simulink model "StandaloneDAQv07_R2014a"  (R2014a)
settings: Solver=FixedStepDiscrete  SolverMode=MultiTasking  StartTime=0.0  StopTime=inf  FixedStep=0.0005  RelTol=1e-3
values from neighbouring files (symbols this model uses):
  ANOMALY_INIT = 10    [DAQParams3_1ms_DDA.m]
  Calibration = getCalibrationParams_ATRIAS()    [DAQParams3_1ms_DDA.m]
  EnableFT = 0    [DAQParams3_1ms_DDA.m]
  EncoderAngleLimits = [60 240; 120 300; 60 240; 120 300; 60 240; 120 300; 60 240; 120 300; -30 30; -30 30; -inf inf; -inf inf; -inf inf; -inf inf; -30 30; -30 30; -inf inf; -90 90; -90 90]*pi/180    [DAQParams3_1ms_DDA.m]
  EncoderFiltSys = getDerivFilter(2, 5, 5, Ts)    [DAQParams3_1ms_DDA.m]
  EncoderThreshold = [5; 5; 5; 5; 5; 5; 5; 5; 5; 5; 250; 250; 250; 250; 5; 5; 5; 5; 5]*pi/180    [DAQParams3_1ms_DDA.m]
  IMUAngleLimits = [-180 180; -90 90; -90 90]*pi/180    [DAQParams3_1ms_DDA.m]
  IMUCommand = 70    [DAQParams3_1ms_DDA.m]
  IMUThreshold = 5*pi/180    (= 0.0872664625997)    [DAQParams3_1ms_DDA.m]
  MAX_ANOMALY = 30    [DAQParams3_1ms_DDA.m]
  MedullaCommand = 0    [DAQParams3_1ms_DDA.m]
  MicrostrainFiltSys = getDerivFilter(2, 5, 5, TsMicrostrain)    [DAQParams3_1ms_DDA.m]
  MODBUS_TIMEOUT = 0.02    [DAQParams3_1ms_DDA.m]
  ResetDAQ = 0    [DAQParams3_1ms_DDA.m]
  ResetYaw = 0    [DAQParams3_1ms_DDA.m]
  STREAMING_TIMEOUT = 0.1    [DAQParams3_1ms_DDA.m]
  TareFT = 0    [DAQParams3_1ms_DDA.m]
  Ts = 0.001    [DAQParams3_1ms_DDA.m]
  UseMicrostrainRate = 0    [DAQParams3_1ms_DDA.m]
undefined symbols (not defined in the file or in its folder): FTCalibration, GearOffset, IMUTorsoOffset, m_XR17D15x, standard
libraries: xpcethercatlib x167, speedgoatlib x13, dspswit3 x2, simulink x2, xpcseriallib x1, SpeedgoatModified x1
(part 2 of 4)

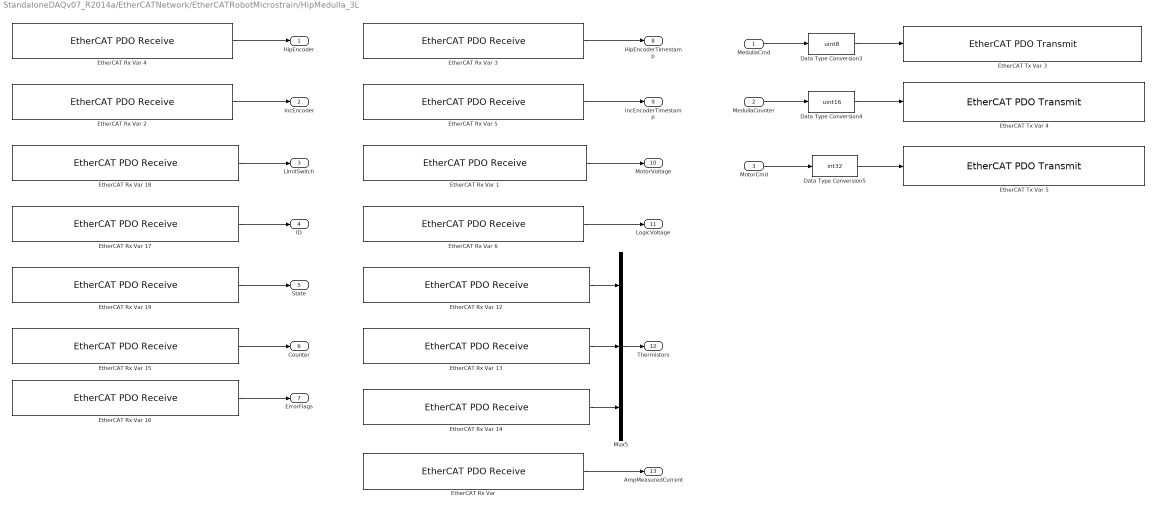
== system StandaloneDAQv07_R2014a/EtherCATNetwork/EtherCATRobotMicrostrain/HipMedulla_3L ==
  MedullaCmd : Inport
  MedullaCounter : Inport  Port=2
  MotorCmd : Inport  Port=3
  Data Type Conversion3 : DataTypeConversion  OutDataTypeStr=uint8  RndMeth=Simplest
  Data Type Conversion4 : DataTypeConversion  OutDataTypeStr=uint16  RndMeth=Simplest
  Data Type Conversion5 : DataTypeConversion  OutDataTypeStr=int32  RndMeth=Simplest
  "EtherCAT Rx Var " : xpcethercatlib/EtherCAT PDO Receive  Priority=2  sig_name=Box 6 (ATRIAS 2.1 Hip (Medulla 1.5)).Measured Current.Amp Measured Current  sig_offset=2480  sig_type=int16  type_size=16  sig_dim=1  device_id=0  sample_time=0.000500
  EtherCAT Rx Var 1 : xpcethercatlib/EtherCAT PDO Receive  Priority=2  sig_name=Box 6 (ATRIAS 2.1 Hip (Medulla 1.5)).Power.Motor Voltage  sig_offset=2400  sig_type=uint16  type_size=16  sig_dim=1  device_id=0  sample_time=0.000500
  EtherCAT Rx Var 12 : xpcethercatlib/EtherCAT PDO Receive  Priority=2  sig_name=Box 6 (ATRIAS 2.1 Hip (Medulla 1.5)).Thermistors.Thermistor 0  sig_offset=2432  sig_type=uint16  type_size=16  sig_dim=1  device_id=0  sample_time=0.000500
  EtherCAT Rx Var 13 : xpcethercatlib/EtherCAT PDO Receive  Priority=2  sig_name=Box 6 (ATRIAS 2.1 Hip (Medulla 1.5)).Thermistors.Thermistor 1  sig_offset=2448  sig_type=uint16  type_size=16  sig_dim=1  device_id=0  sample_time=0.000500
  EtherCAT Rx Var 14 : xpcethercatlib/EtherCAT PDO Receive  Priority=2  sig_name=Box 6 (ATRIAS 2.1 Hip (Medulla 1.5)).Thermistors.Thermistor 2  sig_offset=2464  sig_type=uint16  type_size=16  sig_dim=1  device_id=0  sample_time=0.000500
  EtherCAT Rx Var 15 : xpcethercatlib/EtherCAT PDO Receive  Priority=2  sig_name=Box 6 (ATRIAS 2.1 Hip (Medulla 1.5)).uController Status.Counter  sig_offset=2328  sig_type=uint8  type_size=8  sig_dim=1  device_id=0  sample_time=0.000500
  EtherCAT Rx Var 16 : xpcethercatlib/EtherCAT PDO Receive  Priority=2  sig_name=Box 6 (ATRIAS 2.1 Hip (Medulla 1.5)).uController Status.Error Flags  sig_offset=2336  sig_type=uint8  type_size=8  sig_dim=1  device_id=0  sample_time=0.000500
  EtherCAT Rx Var 17 : xpcethercatlib/EtherCAT PDO Receive  Priority=2  sig_name=Box 6 (ATRIAS 2.1 Hip (Medulla 1.5)).uController Status.ID  sig_offset=2312  sig_type=uint8  type_size=8  sig_dim=1  device_id=0  sample_time=0.000500
  EtherCAT Rx Var 18 : xpcethercatlib/EtherCAT PDO Receive  Priority=2  sig_name=Box 6 (ATRIAS 2.1 Hip (Medulla 1.5)).uController Status.Limit Switch  sig_offset=2344  sig_type=uint8  type_size=8  sig_dim=1  device_id=0  sample_time=0.000500
  EtherCAT Rx Var 19 : xpcethercatlib/EtherCAT PDO Receive  Priority=2  sig_name=Box 6 (ATRIAS 2.1 Hip (Medulla 1.5)).uController Status.State  sig_offset=2320  sig_type=uint8  type_size=8  sig_dim=1  device_id=0  sample_time=0.000500
  EtherCAT Rx Var 2 : xpcethercatlib/EtherCAT PDO Receive  Priority=2  sig_name=Box 6 (ATRIAS 2.1 Hip (Medulla 1.5)).Incremental Encoder.Incremental Encoder  sig_offset=2496  sig_type=uint16  type_size=16  sig_dim=1  device_id=0  sample_time=0.000500
  EtherCAT Rx Var 3 : xpcethercatlib/EtherCAT PDO Receive  Priority=2  sig_name=Box 6 (ATRIAS 2.1 Hip (Medulla 1.5)).Hip Encoder.Timestamp  sig_offset=2384  sig_type=uint16  type_size=16  sig_dim=1  device_id=0  sample_time=0.000500
  EtherCAT Rx Var 4 : xpcethercatlib/EtherCAT PDO Receive  Priority=2  sig_name=Box 6 (ATRIAS 2.1 Hip (Medulla 1.5)).Hip Encoder.Encoder  sig_offset=2352  sig_type=uint32  type_size=32  sig_dim=1  device_id=0  sample_time=0.000500
  EtherCAT Rx Var 5 : xpcethercatlib/EtherCAT PDO Receive  Priority=2  sig_name=Box 6 (ATRIAS 2.1 Hip (Medulla 1.5)).Incremental Encoder.Incremental Encoder Timestamp  sig_offset=2512  sig_type=uint16  type_size=16  sig_dim=1  device_id=0  sample_time=0.000500
  EtherCAT Rx Var 6 : xpcethercatlib/EtherCAT PDO Receive  Priority=2  sig_name=Box 6 (ATRIAS 2.1 Hip (Medulla 1.5)).Power.Logic Voltage  sig_offset=2416  sig_type=uint16  type_size=16  sig_dim=1  device_id=0  sample_time=0.000500
  EtherCAT Tx Var 3 : xpcethercatlib/EtherCAT PDO Transmit   Priority=3  sig_name=Box 6 (ATRIAS 2.1 Hip (Medulla 1.5)).uControllerInput.Command  sig_offset=2312  sig_type=uint8  type_size=8  sig_dim=1  device_id=0  sample_time=0.000500
  EtherCAT Tx Var 4 : xpcethercatlib/EtherCAT PDO Transmit   Priority=3  sig_name=Box 6 (ATRIAS 2.1 Hip (Medulla 1.5)).uControllerInput.Counter  sig_offset=2320  sig_type=uint16  type_size=16  sig_dim=1  device_id=0  sample_time=0.000500
  EtherCAT Tx Var 5 : xpcethercatlib/EtherCAT PDO Transmit   Priority=3  sig_name=Box 6 (ATRIAS 2.1 Hip (Medulla 1.5)).uControllerInput.Motor Current  sig_offset=2336  sig_type=int32  type_size=32  sig_dim=1  device_id=0  sample_time=0.000500
  Mux5 : Mux  Inputs=3
  HipEncoder : Outport
  IncEncoder : Outport  Port=2
  LimitSwitch : Outport  Port=3
  ID : Outport  Port=4
  State : Outport  Port=5
  Counter : Outport  Port=6
  ErrorFlags : Outport  Port=7
  HipEncoderTimestamp : Outport  Port=8
  IncEncoderTimestamp : Outport  Port=9
  MotorVoltage : Outport  Port=10
  LogicVoltage : Outport  Port=11
  Thermistors : Outport  Port=12
  AmpMeasuredCurrent : Outport  Port=13
  wires:
  Data Type Conversion3/1 -> EtherCAT Tx Var 3/1
  Data Type Conversion4/1 -> EtherCAT Tx Var 4/1
  Data Type Conversion5/1 -> EtherCAT Tx Var 5/1
  MedullaCmd/1 -> Data Type Conversion3/1
  MedullaCounter/1 -> Data Type Conversion4/1
  MotorCmd/1 -> Data Type Conversion5/1
  EtherCAT Rx Var 5/1 -> IncEncoderTimestamp/1
  EtherCAT Rx Var 4/1 -> HipEncoder/1
  EtherCAT Rx Var 3/1 -> HipEncoderTimestamp/1
  EtherCAT Rx Var 2/1 -> IncEncoder/1
  EtherCAT Rx Var 15/1 -> Counter/1
  EtherCAT Rx Var 17/1 -> ID/1
  EtherCAT Rx Var 18/1 -> LimitSwitch/1
  EtherCAT Rx Var 19/1 -> State/1
  EtherCAT Rx Var 16/1 -> ErrorFlags/1
  EtherCAT Rx Var 6/1 -> LogicVoltage/1
  EtherCAT Rx Var 1/1 -> MotorVoltage/1
  EtherCAT Rx Var 12/1 -> Mux5/1
  EtherCAT Rx Var 13/1 -> Mux5/2
  EtherCAT Rx Var 14/1 -> Mux5/3
  "EtherCAT Rx Var "/1 -> AmpMeasuredCurrent/1
  Mux5/1 -> Thermistors/1

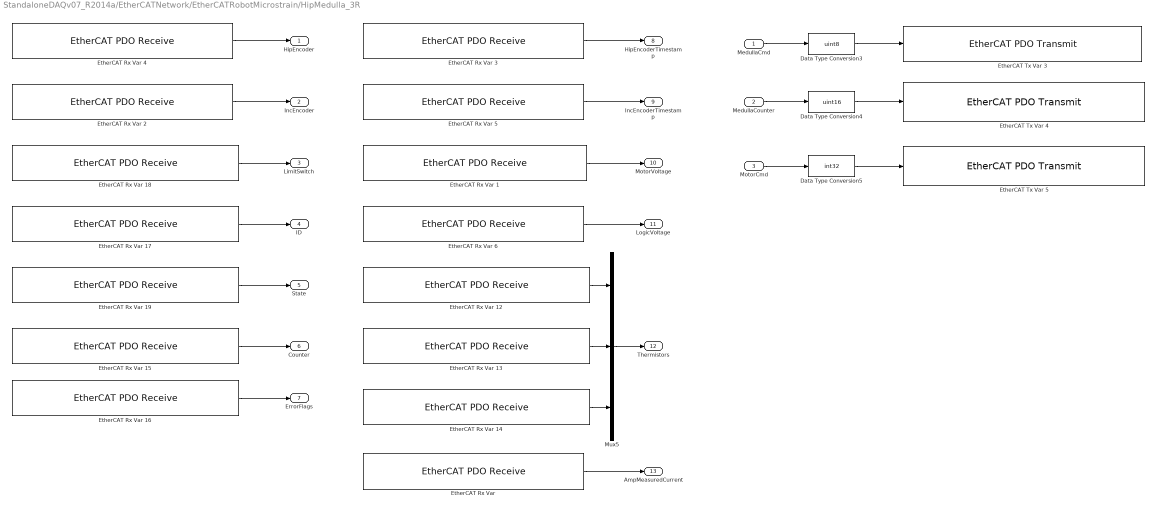
== system StandaloneDAQv07_R2014a/EtherCATNetwork/EtherCATRobotMicrostrain/HipMedulla_3R ==
  MedullaCmd : Inport
  MedullaCounter : Inport  Port=2
  MotorCmd : Inport  Port=3
  Data Type Conversion3 : DataTypeConversion  OutDataTypeStr=uint8  RndMeth=Simplest
  Data Type Conversion4 : DataTypeConversion  OutDataTypeStr=uint16  RndMeth=Simplest
  Data Type Conversion5 : DataTypeConversion  OutDataTypeStr=int32  RndMeth=Simplest
  "EtherCAT Rx Var " : xpcethercatlib/EtherCAT PDO Receive  Priority=2  sig_name=Box 5 (ATRIAS 2.1 Hip (Medulla 1.5)).Measured Current.Amp Measured Current  sig_offset=2264  sig_type=int16  type_size=16  sig_dim=1  device_id=0  sample_time=0.000500
  EtherCAT Rx Var 1 : xpcethercatlib/EtherCAT PDO Receive  Priority=2  sig_name=Box 5 (ATRIAS 2.1 Hip (Medulla 1.5)).Power.Motor Voltage  sig_offset=2184  sig_type=uint16  type_size=16  sig_dim=1  device_id=0  sample_time=0.000500
  EtherCAT Rx Var 12 : xpcethercatlib/EtherCAT PDO Receive  Priority=2  sig_name=Box 5 (ATRIAS 2.1 Hip (Medulla 1.5)).Thermistors.Thermistor 0  sig_offset=2216  sig_type=uint16  type_size=16  sig_dim=1  device_id=0  sample_time=0.000500
  EtherCAT Rx Var 13 : xpcethercatlib/EtherCAT PDO Receive  Priority=2  sig_name=Box 5 (ATRIAS 2.1 Hip (Medulla 1.5)).Thermistors.Thermistor 1  sig_offset=2232  sig_type=uint16  type_size=16  sig_dim=1  device_id=0  sample_time=0.000500
  EtherCAT Rx Var 14 : xpcethercatlib/EtherCAT PDO Receive  Priority=2  sig_name=Box 5 (ATRIAS 2.1 Hip (Medulla 1.5)).Thermistors.Thermistor 2  sig_offset=2248  sig_type=uint16  type_size=16  sig_dim=1  device_id=0  sample_time=0.000500
  EtherCAT Rx Var 15 : xpcethercatlib/EtherCAT PDO Receive  Priority=2  sig_name=Box 5 (ATRIAS 2.1 Hip (Medulla 1.5)).uController Status.Counter  sig_offset=2112  sig_type=uint8  type_size=8  sig_dim=1  device_id=0  sample_time=0.000500
  EtherCAT Rx Var 16 : xpcethercatlib/EtherCAT PDO Receive  Priority=2  sig_name=Box 5 (ATRIAS 2.1 Hip (Medulla 1.5)).uController Status.Error Flags  sig_offset=2120  sig_type=uint8  type_size=8  sig_dim=1  device_id=0  sample_time=0.000500
  EtherCAT Rx Var 17 : xpcethercatlib/EtherCAT PDO Receive  Priority=2  sig_name=Box 5 (ATRIAS 2.1 Hip (Medulla 1.5)).uController Status.ID  sig_offset=2096  sig_type=uint8  type_size=8  sig_dim=1  device_id=0  sample_time=0.000500
  EtherCAT Rx Var 18 : xpcethercatlib/EtherCAT PDO Receive  Priority=2  sig_name=Box 5 (ATRIAS 2.1 Hip (Medulla 1.5)).uController Status.Limit Switch  sig_offset=2128  sig_type=uint8  type_size=8  sig_dim=1  device_id=0  sample_time=0.000500
  EtherCAT Rx Var 19 : xpcethercatlib/EtherCAT PDO Receive  Priority=2  sig_name=Box 5 (ATRIAS 2.1 Hip (Medulla 1.5)).uController Status.State  sig_offset=2104  sig_type=uint8  type_size=8  sig_dim=1  device_id=0  sample_time=0.000500
  EtherCAT Rx Var 2 : xpcethercatlib/EtherCAT PDO Receive  Priority=2  sig_name=Box 5 (ATRIAS 2.1 Hip (Medulla 1.5)).Incremental Encoder.Incremental Encoder  sig_offset=2280  sig_type=uint16  type_size=16  sig_dim=1  device_id=0  sample_time=0.000500
  EtherCAT Rx Var 3 : xpcethercatlib/EtherCAT PDO Receive  Priority=2  sig_name=Box 5 (ATRIAS 2.1 Hip (Medulla 1.5)).Hip Encoder.Timestamp  sig_offset=2168  sig_type=uint16  type_size=16  sig_dim=1  device_id=0  sample_time=0.000500
  EtherCAT Rx Var 4 : xpcethercatlib/EtherCAT PDO Receive  Priority=2  sig_name=Box 5 (ATRIAS 2.1 Hip (Medulla 1.5)).Hip Encoder.Encoder  sig_offset=2136  sig_type=uint32  type_size=32  sig_dim=1  device_id=0  sample_time=0.000500
  EtherCAT Rx Var 5 : xpcethercatlib/EtherCAT PDO Receive  Priority=2  sig_name=Box 5 (ATRIAS 2.1 Hip (Medulla 1.5)).Incremental Encoder.Incremental Encoder Timestamp  sig_offset=2296  sig_type=uint16  type_size=16  sig_dim=1  device_id=0  sample_time=0.000500
  EtherCAT Rx Var 6 : xpcethercatlib/EtherCAT PDO Receive  Priority=2  sig_name=Box 5 (ATRIAS 2.1 Hip (Medulla 1.5)).Power.Logic Voltage  sig_offset=2200  sig_type=uint16  type_size=16  sig_dim=1  device_id=0  sample_time=0.000500
  EtherCAT Tx Var 3 : xpcethercatlib/EtherCAT PDO Transmit   Priority=3  sig_name=Box 5 (ATRIAS 2.1 Hip (Medulla 1.5)).uControllerInput.Command  sig_offset=2096  sig_type=uint8  type_size=8  sig_dim=1  device_id=0  sample_time=0.000500
  EtherCAT Tx Var 4 : xpcethercatlib/EtherCAT PDO Transmit   Priority=3  sig_name=Box 5 (ATRIAS 2.1 Hip (Medulla 1.5)).uControllerInput.Counter  sig_offset=2104  sig_type=uint16  type_size=16  sig_dim=1  device_id=0  sample_time=0.000500
  EtherCAT Tx Var 5 : xpcethercatlib/EtherCAT PDO Transmit   Priority=3  sig_name=Box 5 (ATRIAS 2.1 Hip (Medulla 1.5)).uControllerInput.Motor Current  sig_offset=2120  sig_type=int32  type_size=32  sig_dim=1  device_id=0  sample_time=0.000500
  Mux5 : Mux  Inputs=3
  HipEncoder : Outport
  IncEncoder : Outport  Port=2
  LimitSwitch : Outport  Port=3
  ID : Outport  Port=4
  State : Outport  Port=5
  Counter : Outport  Port=6
  ErrorFlags : Outport  Port=7
  HipEncoderTimestamp : Outport  Port=8
  IncEncoderTimestamp : Outport  Port=9
  MotorVoltage : Outport  Port=10
  LogicVoltage : Outport  Port=11
  Thermistors : Outport  Port=12
  AmpMeasuredCurrent : Outport  Port=13
  wires:
  Data Type Conversion3/1 -> EtherCAT Tx Var 3/1
  Data Type Conversion4/1 -> EtherCAT Tx Var 4/1
  Data Type Conversion5/1 -> EtherCAT Tx Var 5/1
  MedullaCmd/1 -> Data Type Conversion3/1
  MedullaCounter/1 -> Data Type Conversion4/1
  MotorCmd/1 -> Data Type Conversion5/1
  EtherCAT Rx Var 5/1 -> IncEncoderTimestamp/1
  EtherCAT Rx Var 4/1 -> HipEncoder/1
  EtherCAT Rx Var 3/1 -> HipEncoderTimestamp/1
  EtherCAT Rx Var 2/1 -> IncEncoder/1
  EtherCAT Rx Var 15/1 -> Counter/1
  EtherCAT Rx Var 17/1 -> ID/1
  EtherCAT Rx Var 18/1 -> LimitSwitch/1
  EtherCAT Rx Var 19/1 -> State/1
  EtherCAT Rx Var 16/1 -> ErrorFlags/1
  EtherCAT Rx Var 6/1 -> LogicVoltage/1
  EtherCAT Rx Var 1/1 -> MotorVoltage/1
  EtherCAT Rx Var 12/1 -> Mux5/1
  EtherCAT Rx Var 13/1 -> Mux5/2
  EtherCAT Rx Var 14/1 -> Mux5/3
  "EtherCAT Rx Var "/1 -> AmpMeasuredCurrent/1
  Mux5/1 -> Thermistors/1

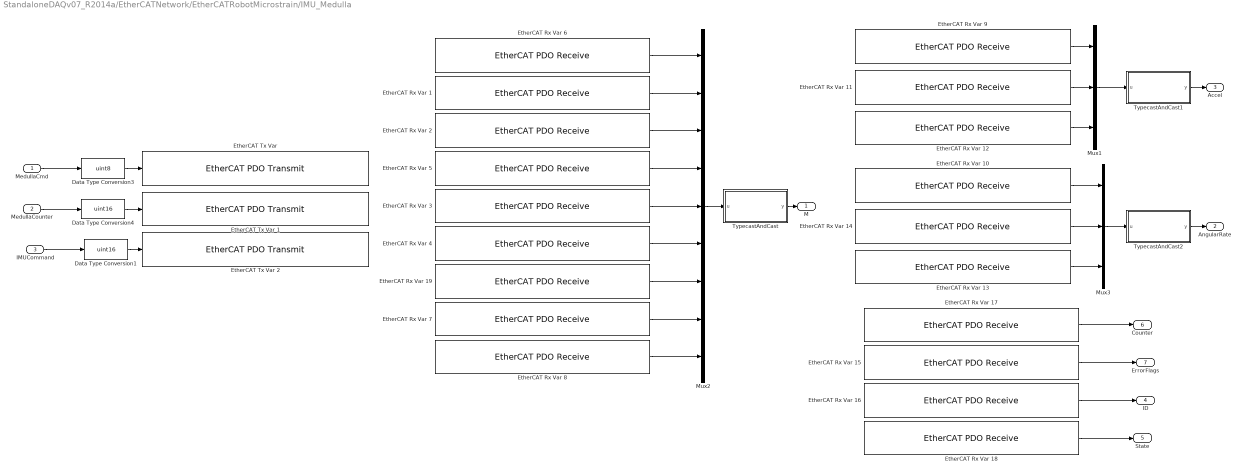
== system StandaloneDAQv07_R2014a/EtherCATNetwork/EtherCATRobotMicrostrain/IMU_Medulla ==
  MedullaCmd : Inport
  MedullaCounter : Inport  Port=2
  IMUCommand : Inport  Port=3
  Data Type Conversion1 : DataTypeConversion  OutDataTypeStr=uint16  RndMeth=Simplest
  Data Type Conversion3 : DataTypeConversion  OutDataTypeStr=uint8  RndMeth=Simplest
  Data Type Conversion4 : DataTypeConversion  OutDataTypeStr=uint16  RndMeth=Simplest
  EtherCAT Rx Var 1 : xpcethercatlib/EtherCAT PDO Receive  Priority=2  sig_name=Box 7 (ATRIAS 2.1 Microstrain IMU (Medulla 1.5)).M.M12  sig_offset=2784  sig_type=uint32  type_size=32  sig_dim=1  device_id=0  sample_time=0.000500
  EtherCAT Rx Var 10 : xpcethercatlib/EtherCAT PDO Receive  Priority=2  sig_name=Box 7 (ATRIAS 2.1 Microstrain IMU (Medulla 1.5)).Xaxes.XAngRate  sig_offset=2560  sig_type=uint32  type_size=32  sig_dim=1  device_id=0  sample_time=0.000500
  EtherCAT Rx Var 11 : xpcethercatlib/EtherCAT PDO Receive  Priority=2  sig_name=Box 7 (ATRIAS 2.1 Microstrain IMU (Medulla 1.5)).Yaxes.YAccel  sig_offset=2656  sig_type=uint32  type_size=32  sig_dim=1  device_id=0  sample_time=0.000500
  EtherCAT Rx Var 12 : xpcethercatlib/EtherCAT PDO Receive  Priority=2  sig_name=Box 7 (ATRIAS 2.1 Microstrain IMU (Medulla 1.5)).Zaxes.ZAccel  sig_offset=2720  sig_type=uint32  type_size=32  sig_dim=1  device_id=0  sample_time=0.000500
  EtherCAT Rx Var 13 : xpcethercatlib/EtherCAT PDO Receive  Priority=2  sig_name=Box 7 (ATRIAS 2.1 Microstrain IMU (Medulla 1.5)).Zaxes.ZAngRate  sig_offset=2688  sig_type=uint32  type_size=32  sig_dim=1  device_id=0  sample_time=0.000500
  EtherCAT Rx Var 14 : xpcethercatlib/EtherCAT PDO Receive  Priority=2  sig_name=Box 7 (ATRIAS 2.1 Microstrain IMU (Medulla 1.5)).Yaxes.YAngRate  sig_offset=2624  sig_type=uint32  type_size=32  sig_dim=1  device_id=0  sample_time=0.000500
  EtherCAT Rx Var 15 : xpcethercatlib/EtherCAT PDO Receive  Priority=2  sig_name=Box 7 (ATRIAS 2.1 Microstrain IMU (Medulla 1.5)).uController Status.Error Flags  sig_offset=2552  sig_type=uint8  type_size=8  sig_dim=1  device_id=0  sample_time=0.000500
  EtherCAT Rx Var 16 : xpcethercatlib/EtherCAT PDO Receive  Priority=2  sig_name=Box 7 (ATRIAS 2.1 Microstrain IMU (Medulla 1.5)).uController Status.ID  sig_offset=2528  sig_type=uint8  type_size=8  sig_dim=1  device_id=0  sample_time=0.000500
  EtherCAT Rx Var 17 : xpcethercatlib/EtherCAT PDO Receive  Priority=2  sig_name=Box 7 (ATRIAS 2.1 Microstrain IMU (Medulla 1.5)).uController Status.Counter  sig_offset=2544  sig_type=uint8  type_size=8  sig_dim=1  device_id=0  sample_time=0.000500
  EtherCAT Rx Var 18 : xpcethercatlib/EtherCAT PDO Receive  Priority=2  sig_name=Box 7 (ATRIAS 2.1 Microstrain IMU (Medulla 1.5)).uController Status.State  sig_offset=2536  sig_type=uint8  type_size=8  sig_dim=1  device_id=0  sample_time=0.000500
  EtherCAT Rx Var 19 : xpcethercatlib/EtherCAT PDO Receive  Priority=2  sig_name=Box 7 (ATRIAS 2.1 Microstrain IMU (Medulla 1.5)).M.M31  sig_offset=2944  sig_type=uint32  type_size=32  sig_dim=1  device_id=0  sample_time=0.000500
  EtherCAT Rx Var 2 : xpcethercatlib/EtherCAT PDO Receive  Priority=2  sig_name=Box 7 (ATRIAS 2.1 Microstrain IMU (Medulla 1.5)).M.M13  sig_offset=2816  sig_type=uint32  type_size=32  sig_dim=1  device_id=0  sample_time=0.000500
  EtherCAT Rx Var 3 : xpcethercatlib/EtherCAT PDO Receive  Priority=2  sig_name=Box 7 (ATRIAS 2.1 Microstrain IMU (Medulla 1.5)).M.M22  sig_offset=2880  sig_type=uint32  type_size=32  sig_dim=1  device_id=0  sample_time=0.000500
  EtherCAT Rx Var 4 : xpcethercatlib/EtherCAT PDO Receive  Priority=2  sig_name=Box 7 (ATRIAS 2.1 Microstrain IMU (Medulla 1.5)).M.M23  sig_offset=2912  sig_type=uint32  type_size=32  sig_dim=1  device_id=0  sample_time=0.000500
  EtherCAT Rx Var 5 : xpcethercatlib/EtherCAT PDO Receive  Priority=2  sig_name=Box 7 (ATRIAS 2.1 Microstrain IMU (Medulla 1.5)).M.M21  sig_offset=2848  sig_type=uint32  type_size=32  sig_dim=1  device_id=0  sample_time=0.000500
  EtherCAT Rx Var 6 : xpcethercatlib/EtherCAT PDO Receive  Priority=2  sig_name=Box 7 (ATRIAS 2.1 Microstrain IMU (Medulla 1.5)).M.M11  sig_offset=2752  sig_type=uint32  type_size=32  sig_dim=1  device_id=0  sample_time=0.000500
  EtherCAT Rx Var 7 : xpcethercatlib/EtherCAT PDO Receive  Priority=2  sig_name=Box 7 (ATRIAS 2.1 Microstrain IMU (Medulla 1.5)).M.M32  sig_offset=2976  sig_type=uint32  type_size=32  sig_dim=1  device_id=0  sample_time=0.000500
  EtherCAT Rx Var 8 : xpcethercatlib/EtherCAT PDO Receive  Priority=2  sig_name=Box 7 (ATRIAS 2.1 Microstrain IMU (Medulla 1.5)).M.M33  sig_offset=3008  sig_type=uint32  type_size=32  sig_dim=1  device_id=0  sample_time=0.000500
  EtherCAT Rx Var 9 : xpcethercatlib/EtherCAT PDO Receive  Priority=2  sig_name=Box 7 (ATRIAS 2.1 Microstrain IMU (Medulla 1.5)).Xaxes.XAccel  sig_offset=2592  sig_type=uint32  type_size=32  sig_dim=1  device_id=0  sample_time=0.000500
  "EtherCAT Tx Var " : xpcethercatlib/EtherCAT PDO Transmit   Priority=3  sig_name=Box 7 (ATRIAS 2.1 Microstrain IMU (Medulla 1.5)).uControllerInput.Command  sig_offset=2528  sig_type=uint8  type_size=8  sig_dim=1  device_id=0  sample_time=0.000500
  EtherCAT Tx Var 1 : xpcethercatlib/EtherCAT PDO Transmit   Priority=3  sig_name=Box 7 (ATRIAS 2.1 Microstrain IMU (Medulla 1.5)).uControllerInput.Counter  sig_offset=2536  sig_type=uint16  type_size=16  sig_dim=1  device_id=0  sample_time=0.000500
  EtherCAT Tx Var 2 : xpcethercatlib/EtherCAT PDO Transmit   Priority=3  sig_name=Box 7 (ATRIAS 2.1 Microstrain IMU (Medulla 1.5)).uControllerInput.IMU_cmd  sig_offset=2552  sig_type=uint16  type_size=16  sig_dim=1  device_id=0  sample_time=0.000500
  Mux1 : Mux  Inputs=3
  Mux2 : Mux  Inputs=9
  Mux3 : Mux  Inputs=3
  TypecastAndCast : MATLAB Function  TreatAsAtomicUnit=on
  TypecastAndCast1 : MATLAB Function  TreatAsAtomicUnit=on
  TypecastAndCast2 : MATLAB Function  TreatAsAtomicUnit=on
  M : Outport
  AngularRate : Outport  Port=2
  Accel : Outport  Port=3
  ID : Outport  Port=4
  State : Outport  Port=5
  Counter : Outport  Port=6
  ErrorFlags : Outport  Port=7
  wires:
  Data Type Conversion3/1 -> "EtherCAT Tx Var "/1
  Data Type Conversion4/1 -> EtherCAT Tx Var 1/1
  MedullaCmd/1 -> Data Type Conversion3/1
  MedullaCounter/1 -> Data Type Conversion4/1
  IMUCommand/1 -> Data Type Conversion1/1
  Data Type Conversion1/1 -> EtherCAT Tx Var 2/1
  EtherCAT Rx Var 17/1 -> Counter/1
  EtherCAT Rx Var 15/1 -> ErrorFlags/1
  EtherCAT Rx Var 16/1 -> ID/1
  EtherCAT Rx Var 18/1 -> State/1
  EtherCAT Rx Var 13/1 -> Mux3/3
  EtherCAT Rx Var 14/1 -> Mux3/2
  EtherCAT Rx Var 10/1 -> Mux3/1
  EtherCAT Rx Var 12/1 -> Mux1/3
  EtherCAT Rx Var 11/1 -> Mux1/2
  EtherCAT Rx Var 9/1 -> Mux1/1
  Mux1/1 -> TypecastAndCast1/1(u)
  Mux3/1 -> TypecastAndCast2/1(u)
  Mux2/1 -> TypecastAndCast/1(u)
  TypecastAndCast/1(y) -> M/1
  TypecastAndCast1/1(y) -> Accel/1
  TypecastAndCast2/1(y) -> AngularRate/1
  EtherCAT Rx Var 1/1 -> Mux2/2
  EtherCAT Rx Var 19/1 -> Mux2/7
  EtherCAT Rx Var 2/1 -> Mux2/3
  EtherCAT Rx Var 3/1 -> Mux2/5
  EtherCAT Rx Var 4/1 -> Mux2/6
  EtherCAT Rx Var 5/1 -> Mux2/4
  EtherCAT Rx Var 6/1 -> Mux2/1
  EtherCAT Rx Var 7/1 -> Mux2/8
  EtherCAT Rx Var 8/1 -> Mux2/9

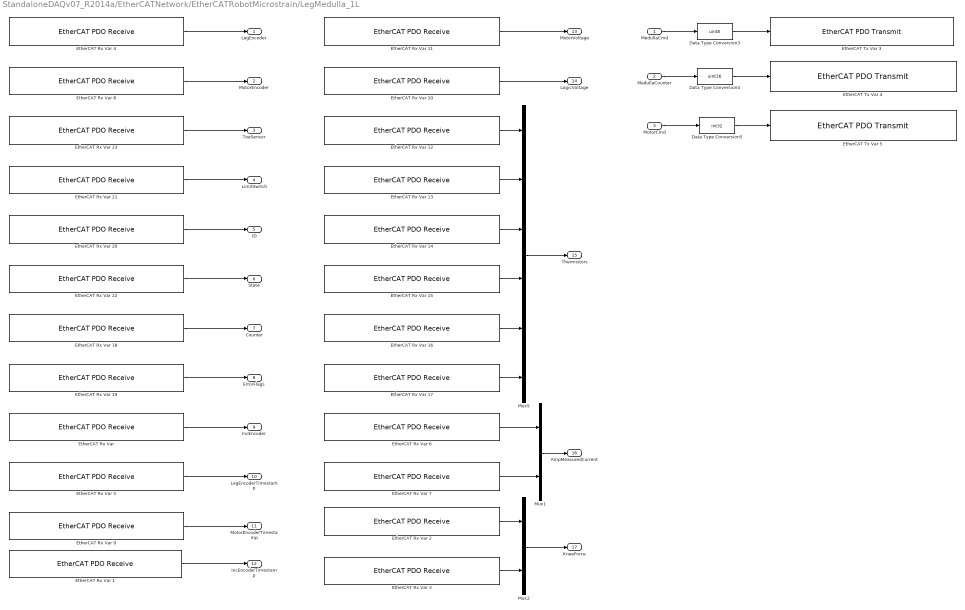
== system StandaloneDAQv07_R2014a/EtherCATNetwork/EtherCATRobotMicrostrain/LegMedulla_1L ==
  MedullaCmd : Inport
  MedullaCounter : Inport  Port=2
  MotorCmd : Inport  Port=3
  Data Type Conversion3 : DataTypeConversion  OutDataTypeStr=uint8  RndMeth=Simplest
  Data Type Conversion4 : DataTypeConversion  OutDataTypeStr=uint16  RndMeth=Simplest
  Data Type Conversion5 : DataTypeConversion  OutDataTypeStr=int32  RndMeth=Simplest
  "EtherCAT Rx Var " : xpcethercatlib/EtherCAT PDO Receive  Priority=2  sig_name=Box 1 (ATRIAS 2.1 Leg (Medulla 1.5)).Incremental Encoder.Incremental Encoder  sig_offset=744  sig_type=uint16  type_size=16  sig_dim=1  device_id=0  sample_time=0.000500
  EtherCAT Rx Var 1 : xpcethercatlib/EtherCAT PDO Receive  Priority=2  sig_name=Box 1 (ATRIAS 2.1 Leg (Medulla 1.5)).Incremental Encoder.Incremental Encoder Timestamp  sig_offset=760  sig_type=uint16  type_size=16  sig_dim=1  device_id=0  sample_time=0.000500
  EtherCAT Rx Var 10 : xpcethercatlib/EtherCAT PDO Receive  Priority=2  sig_name=Box 1 (ATRIAS 2.1 Leg (Medulla 1.5)).Power.Logic Voltage  sig_offset=792  sig_type=uint16  type_size=16  sig_dim=1  device_id=0  sample_time=0.000500
  EtherCAT Rx Var 11 : xpcethercatlib/EtherCAT PDO Receive  Priority=2  sig_name=Box 1 (ATRIAS 2.1 Leg (Medulla 1.5)).Power.Motor Voltage  sig_offset=776  sig_type=uint16  type_size=16  sig_dim=1  device_id=0  sample_time=0.000500
  EtherCAT Rx Var 12 : xpcethercatlib/EtherCAT PDO Receive  Priority=2  sig_name=Box 1 (ATRIAS 2.1 Leg (Medulla 1.5)).Thermistors.Thermistor 0  sig_offset=808  sig_type=uint16  type_size=16  sig_dim=1  device_id=0  sample_time=0.000500
  EtherCAT Rx Var 13 : xpcethercatlib/EtherCAT PDO Receive  Priority=2  sig_name=Box 1 (ATRIAS 2.1 Leg (Medulla 1.5)).Thermistors.Thermistor 1  sig_offset=824  sig_type=uint16  type_size=16  sig_dim=1  device_id=0  sample_time=0.000500
  EtherCAT Rx Var 14 : xpcethercatlib/EtherCAT PDO Receive  Priority=2  sig_name=Box 1 (ATRIAS 2.1 Leg (Medulla 1.5)).Thermistors.Thermistor 2  sig_offset=840  sig_type=uint16  type_size=16  sig_dim=1  device_id=0  sample_time=0.000500
  EtherCAT Rx Var 15 : xpcethercatlib/EtherCAT PDO Receive  Priority=2  sig_name=Box 1 (ATRIAS 2.1 Leg (Medulla 1.5)).Thermistors.Thermistor 3  sig_offset=856  sig_type=uint16  type_size=16  sig_dim=1  device_id=0  sample_time=0.000500
  EtherCAT Rx Var 16 : xpcethercatlib/EtherCAT PDO Receive  Priority=2  sig_name=Box 1 (ATRIAS 2.1 Leg (Medulla 1.5)).Thermistors.Thermistor 4  sig_offset=872  sig_type=uint16  type_size=16  sig_dim=1  device_id=0  sample_time=0.000500
  EtherCAT Rx Var 17 : xpcethercatlib/EtherCAT PDO Receive  Priority=2  sig_name=Box 1 (ATRIAS 2.1 Leg (Medulla 1.5)).Thermistors.Thermistor 5  sig_offset=888  sig_type=uint16  type_size=16  sig_dim=1  device_id=0  sample_time=0.000500
  EtherCAT Rx Var 18 : xpcethercatlib/EtherCAT PDO Receive  Priority=2  sig_name=Box 1 (ATRIAS 2.1 Leg (Medulla 1.5)).uController Status.Counter  sig_offset=608  sig_type=uint8  type_size=8  sig_dim=1  device_id=0  sample_time=0.000500
  EtherCAT Rx Var 19 : xpcethercatlib/EtherCAT PDO Receive  Priority=2  sig_name=Box 1 (ATRIAS 2.1 Leg (Medulla 1.5)).uController Status.Error Flags  sig_offset=616  sig_type=uint8  type_size=8  sig_dim=1  device_id=0  sample_time=0.000500
  EtherCAT Rx Var 2 : xpcethercatlib/EtherCAT PDO Receive  Priority=2  sig_name=Box 1 (ATRIAS 2.1 Leg (Medulla 1.5)).Knee Force.Knee Force 1  sig_offset=936  sig_type=uint16  type_size=16  sig_dim=1  device_id=0  sample_time=0.000500
  EtherCAT Rx Var 20 : xpcethercatlib/EtherCAT PDO Receive  Priority=2  sig_name=Box 1 (ATRIAS 2.1 Leg (Medulla 1.5)).uController Status.ID  sig_offset=592  sig_type=uint8  type_size=8  sig_dim=1  device_id=0  sample_time=0.000500
  EtherCAT Rx Var 21 : xpcethercatlib/EtherCAT PDO Receive  Priority=2  sig_name=Box 1 (ATRIAS 2.1 Leg (Medulla 1.5)).uController Status.Limit Switch  sig_offset=624  sig_type=uint8  type_size=8  sig_dim=1  device_id=0  sample_time=0.000500
  EtherCAT Rx Var 22 : xpcethercatlib/EtherCAT PDO Receive  Priority=2  sig_name=Box 1 (ATRIAS 2.1 Leg (Medulla 1.5)).uController Status.State  sig_offset=600  sig_type=uint8  type_size=8  sig_dim=1  device_id=0  sample_time=0.000500
  EtherCAT Rx Var 23 : xpcethercatlib/EtherCAT PDO Receive  Priority=2  sig_name=Box 1 (ATRIAS 2.1 Leg (Medulla 1.5)).uController Status.Toe Sensor  sig_offset=632  sig_type=uint16  type_size=16  sig_dim=1  device_id=0  sample_time=0.000500
  EtherCAT Rx Var 3 : xpcethercatlib/EtherCAT PDO Receive  Priority=2  sig_name=Box 1 (ATRIAS 2.1 Leg (Medulla 1.5)).Knee Force.Knee Force 2  sig_offset=952  sig_type=uint16  type_size=16  sig_dim=1  device_id=0  sample_time=0.000500
  EtherCAT Rx Var 4 : xpcethercatlib/EtherCAT PDO Receive  Priority=2  sig_name=Box 1 (ATRIAS 2.1 Leg (Medulla 1.5)).Leg Encoder.Leg Encoder  sig_offset=696  sig_type=uint32  type_size=32  sig_dim=1  device_id=0  sample_time=0.000500
  EtherCAT Rx Var 5 : xpcethercatlib/EtherCAT PDO Receive  Priority=2  sig_name=Box 1 (ATRIAS 2.1 Leg (Medulla 1.5)).Leg Encoder.Leg Encoder Timestamp  sig_offset=728  sig_type=uint16  type_size=16  sig_dim=1  device_id=0  sample_time=0.000500
  EtherCAT Rx Var 6 : xpcethercatlib/EtherCAT PDO Receive  Priority=2  sig_name=Box 1 (ATRIAS 2.1 Leg (Medulla 1.5)).Measured Current.Amp 1 Measured Current  sig_offset=904  sig_type=int16  type_size=16  sig_dim=1  device_id=0  sample_time=0.000500
  EtherCAT Rx Var 7 : xpcethercatlib/EtherCAT PDO Receive  Priority=2  sig_name=Box 1 (ATRIAS 2.1 Leg (Medulla 1.5)).Measured Current.Amp 2 Measured Current  sig_offset=920  sig_type=int16  type_size=16  sig_dim=1  device_id=0  sample_time=0.000500
  EtherCAT Rx Var 8 : xpcethercatlib/EtherCAT PDO Receive  Priority=2  sig_name=Box 1 (ATRIAS 2.1 Leg (Medulla 1.5)).Motor Encoder.Motor Encoder  sig_offset=648  sig_type=uint32  type_size=32  sig_dim=1  device_id=0  sample_time=0.000500
  EtherCAT Rx Var 9 : xpcethercatlib/EtherCAT PDO Receive  Priority=2  sig_name=Box 1 (ATRIAS 2.1 Leg (Medulla 1.5)).Motor Encoder.Motor Encoder Timestamp  sig_offset=680  sig_type=uint16  type_size=16  sig_dim=1  device_id=0  sample_time=0.000500
  EtherCAT Tx Var 3 : xpcethercatlib/EtherCAT PDO Transmit   Priority=3  sig_name=Box 1 (ATRIAS 2.1 Leg (Medulla 1.5)).uControllerInput.Command  sig_offset=592  sig_type=uint8  type_size=8  sig_dim=1  device_id=0  sample_time=0.000500
  EtherCAT Tx Var 4 : xpcethercatlib/EtherCAT PDO Transmit   Priority=3  sig_name=Box 1 (ATRIAS 2.1 Leg (Medulla 1.5)).uControllerInput.Counter  sig_offset=600  sig_type=uint16  type_size=16  sig_dim=1  device_id=0  sample_time=0.000500
  EtherCAT Tx Var 5 : xpcethercatlib/EtherCAT PDO Transmit   Priority=3  sig_name=Box 1 (ATRIAS 2.1 Leg (Medulla 1.5)).uControllerInput.Motor Current  sig_offset=616  sig_type=int32  type_size=32  sig_dim=1  device_id=0  sample_time=0.000500
  Mux1 : Mux  Inputs=2
  Mux2 : Mux  Inputs=2
  Mux5 : Mux  Inputs=6
  LegEncoder : Outport
  MotorEncoder : Outport  Port=2
  ToeSensor : Outport  Port=3
  LimitSwitch : Outport  Port=4
  ID : Outport  Port=5
  State : Outport  Port=6
  Counter : Outport  Port=7
  ErrorFlags : Outport  Port=8
  IncEncoder : Outport  Port=9
  LegEncoderTimestamp : Outport  Port=10
  MotorEncoderTimestamp : Outport  Port=11
  IncEncoderTimestamp : Outport  Port=12
  MotorVoltage : Outport  Port=13
  LogicVoltage : Outport  Port=14
  Thermistors : Outport  Port=15
  AmpMeasuredCurrent : Outport  Port=16
  KneeForce : Outport  Port=17
  wires:
  Data Type Conversion3/1 -> EtherCAT Tx Var 3/1
  Data Type Conversion4/1 -> EtherCAT Tx Var 4/1
  Data Type Conversion5/1 -> EtherCAT Tx Var 5/1
  "EtherCAT Rx Var "/1 -> IncEncoder/1
  EtherCAT Rx Var 1/1 -> IncEncoderTimestamp/1
  EtherCAT Rx Var 2/1 -> Mux2/1
  EtherCAT Rx Var 4/1 -> LegEncoder/1
  EtherCAT Rx Var 5/1 -> LegEncoderTimestamp/1
  EtherCAT Rx Var 6/1 -> Mux1/1
  EtherCAT Rx Var 8/1 -> MotorEncoder/1
  EtherCAT Rx Var 9/1 -> MotorEncoderTimestamp/1
  EtherCAT Rx Var 10/1 -> LogicVoltage/1
  EtherCAT Rx Var 11/1 -> MotorVoltage/1
  EtherCAT Rx Var 13/1 -> Mux5/2
  EtherCAT Rx Var 14/1 -> Mux5/3
  EtherCAT Rx Var 15/1 -> Mux5/4
  EtherCAT Rx Var 16/1 -> Mux5/5
  EtherCAT Rx Var 17/1 -> Mux5/6
  EtherCAT Rx Var 18/1 -> Counter/1
  EtherCAT Rx Var 19/1 -> ErrorFlags/1
  EtherCAT Rx Var 20/1 -> ID/1
  EtherCAT Rx Var 21/1 -> LimitSwitch/1
  EtherCAT Rx Var 22/1 -> State/1
  EtherCAT Rx Var 23/1 -> ToeSensor/1
  MedullaCmd/1 -> Data Type Conversion3/1
  MedullaCounter/1 -> Data Type Conversion4/1
  MotorCmd/1 -> Data Type Conversion5/1
  EtherCAT Rx Var 12/1 -> Mux5/1
  Mux5/1 -> Thermistors/1
  Mux1/1 -> AmpMeasuredCurrent/1
  EtherCAT Rx Var 7/1 -> Mux1/2
  EtherCAT Rx Var 3/1 -> Mux2/2
  Mux2/1 -> KneeForce/1

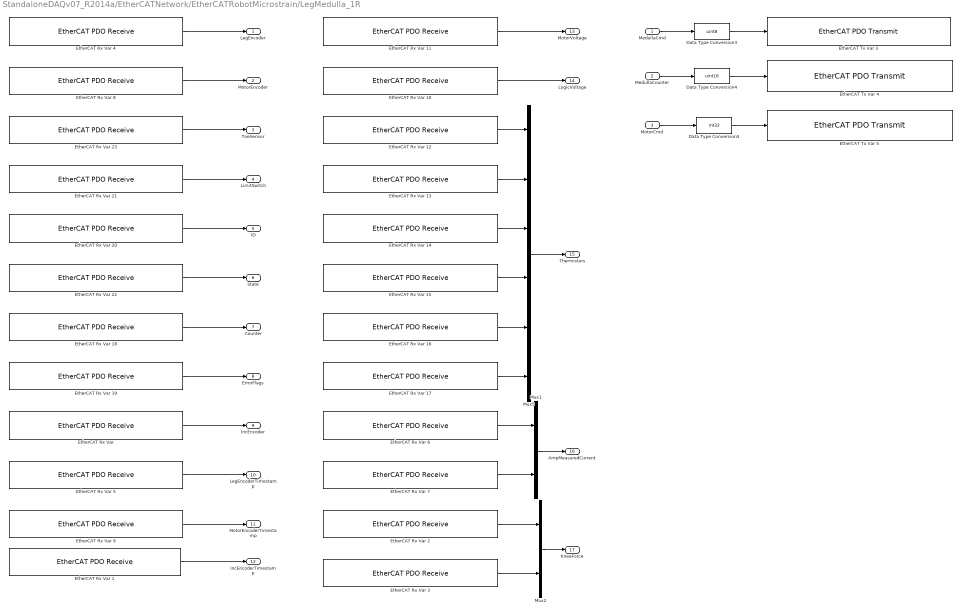
== system StandaloneDAQv07_R2014a/EtherCATNetwork/EtherCATRobotMicrostrain/LegMedulla_1R ==
  MedullaCmd : Inport
  MedullaCounter : Inport  Port=2
  MotorCmd : Inport  Port=3
  Data Type Conversion3 : DataTypeConversion  OutDataTypeStr=uint8  RndMeth=Simplest
  Data Type Conversion4 : DataTypeConversion  OutDataTypeStr=uint16  RndMeth=Simplest
  Data Type Conversion5 : DataTypeConversion  OutDataTypeStr=int32  RndMeth=Simplest
  "EtherCAT Rx Var " : xpcethercatlib/EtherCAT PDO Receive  Priority=2  sig_name=Box 3 (ATRIAS 2.1 Leg (Medulla 1.5)).Incremental Encoder.Incremental Encoder  sig_offset=1496  sig_type=uint16  type_size=16  sig_dim=1  device_id=0  sample_time=0.000500
  EtherCAT Rx Var 1 : xpcethercatlib/EtherCAT PDO Receive  Priority=2  sig_name=Box 3 (ATRIAS 2.1 Leg (Medulla 1.5)).Incremental Encoder.Incremental Encoder Timestamp  sig_offset=1512  sig_type=uint16  type_size=16  sig_dim=1  device_id=0  sample_time=0.000500
  EtherCAT Rx Var 10 : xpcethercatlib/EtherCAT PDO Receive  Priority=2  sig_name=Box 3 (ATRIAS 2.1 Leg (Medulla 1.5)).Power.Logic Voltage  sig_offset=1544  sig_type=uint16  type_size=16  sig_dim=1  device_id=0  sample_time=0.000500
  EtherCAT Rx Var 11 : xpcethercatlib/EtherCAT PDO Receive  Priority=2  sig_name=Box 3 (ATRIAS 2.1 Leg (Medulla 1.5)).Power.Motor Voltage  sig_offset=1528  sig_type=uint16  type_size=16  sig_dim=1  device_id=0  sample_time=0.000500
  EtherCAT Rx Var 12 : xpcethercatlib/EtherCAT PDO Receive  Priority=2  sig_name=Box 3 (ATRIAS 2.1 Leg (Medulla 1.5)).Thermistors.Thermistor 0  sig_offset=1560  sig_type=uint16  type_size=16  sig_dim=1  device_id=0  sample_time=0.000500
  EtherCAT Rx Var 13 : xpcethercatlib/EtherCAT PDO Receive  Priority=2  sig_name=Box 3 (ATRIAS 2.1 Leg (Medulla 1.5)).Thermistors.Thermistor 1  sig_offset=1576  sig_type=uint16  type_size=16  sig_dim=1  device_id=0  sample_time=0.000500
  EtherCAT Rx Var 14 : xpcethercatlib/EtherCAT PDO Receive  Priority=2  sig_name=Box 3 (ATRIAS 2.1 Leg (Medulla 1.5)).Thermistors.Thermistor 2  sig_offset=1592  sig_type=uint16  type_size=16  sig_dim=1  device_id=0  sample_time=0.000500
  EtherCAT Rx Var 15 : xpcethercatlib/EtherCAT PDO Receive  Priority=2  sig_name=Box 3 (ATRIAS 2.1 Leg (Medulla 1.5)).Thermistors.Thermistor 3  sig_offset=1608  sig_type=uint16  type_size=16  sig_dim=1  device_id=0  sample_time=0.000500
  EtherCAT Rx Var 16 : xpcethercatlib/EtherCAT PDO Receive  Priority=2  sig_name=Box 3 (ATRIAS 2.1 Leg (Medulla 1.5)).Thermistors.Thermistor 4  sig_offset=1624  sig_type=uint16  type_size=16  sig_dim=1  device_id=0  sample_time=0.000500
  EtherCAT Rx Var 17 : xpcethercatlib/EtherCAT PDO Receive  Priority=2  sig_name=Box 3 (ATRIAS 2.1 Leg (Medulla 1.5)).Thermistors.Thermistor 5  sig_offset=1640  sig_type=uint16  type_size=16  sig_dim=1  device_id=0  sample_time=0.000500
  EtherCAT Rx Var 18 : xpcethercatlib/EtherCAT PDO Receive  Priority=2  sig_name=Box 3 (ATRIAS 2.1 Leg (Medulla 1.5)).uController Status.Counter  sig_offset=1360  sig_type=uint8  type_size=8  sig_dim=1  device_id=0  sample_time=0.000500
  EtherCAT Rx Var 19 : xpcethercatlib/EtherCAT PDO Receive  Priority=2  sig_name=Box 3 (ATRIAS 2.1 Leg (Medulla 1.5)).uController Status.Error Flags  sig_offset=1368  sig_type=uint8  type_size=8  sig_dim=1  device_id=0  sample_time=0.000500
  EtherCAT Rx Var 2 : xpcethercatlib/EtherCAT PDO Receive  Priority=2  sig_name=Box 3 (ATRIAS 2.1 Leg (Medulla 1.5)).Knee Force.Knee Force 1  sig_offset=1688  sig_type=uint16  type_size=16  sig_dim=1  device_id=0  sample_time=0.000500
  EtherCAT Rx Var 20 : xpcethercatlib/EtherCAT PDO Receive  Priority=2  sig_name=Box 3 (ATRIAS 2.1 Leg (Medulla 1.5)).uController Status.ID  sig_offset=1344  sig_type=uint8  type_size=8  sig_dim=1  device_id=0  sample_time=0.000500
  EtherCAT Rx Var 21 : xpcethercatlib/EtherCAT PDO Receive  Priority=2  sig_name=Box 3 (ATRIAS 2.1 Leg (Medulla 1.5)).uController Status.Limit Switch  sig_offset=1376  sig_type=uint8  type_size=8  sig_dim=1  device_id=0  sample_time=0.000500
  EtherCAT Rx Var 22 : xpcethercatlib/EtherCAT PDO Receive  Priority=2  sig_name=Box 3 (ATRIAS 2.1 Leg (Medulla 1.5)).uController Status.State  sig_offset=1352  sig_type=uint8  type_size=8  sig_dim=1  device_id=0  sample_time=0.000500
  EtherCAT Rx Var 23 : xpcethercatlib/EtherCAT PDO Receive  Priority=2  sig_name=Box 3 (ATRIAS 2.1 Leg (Medulla 1.5)).uController Status.Toe Sensor  sig_offset=1384  sig_type=uint16  type_size=16  sig_dim=1  device_id=0  sample_time=0.000500
  EtherCAT Rx Var 3 : xpcethercatlib/EtherCAT PDO Receive  Priority=2  sig_name=Box 3 (ATRIAS 2.1 Leg (Medulla 1.5)).Knee Force.Knee Force 2  sig_offset=1704  sig_type=uint16  type_size=16  sig_dim=1  device_id=0  sample_time=0.000500
  EtherCAT Rx Var 4 : xpcethercatlib/EtherCAT PDO Receive  Priority=2  sig_name=Box 3 (ATRIAS 2.1 Leg (Medulla 1.5)).Leg Encoder.Leg Encoder  sig_offset=1448  sig_type=uint32  type_size=32  sig_dim=1  device_id=0  sample_time=0.000500
  EtherCAT Rx Var 5 : xpcethercatlib/EtherCAT PDO Receive  Priority=2  sig_name=Box 3 (ATRIAS 2.1 Leg (Medulla 1.5)).Leg Encoder.Leg Encoder Timestamp  sig_offset=1480  sig_type=uint16  type_size=16  sig_dim=1  device_id=0  sample_time=0.000500
  EtherCAT Rx Var 6 : xpcethercatlib/EtherCAT PDO Receive  Priority=2  sig_name=Box 3 (ATRIAS 2.1 Leg (Medulla 1.5)).Measured Current.Amp 1 Measured Current  sig_offset=1656  sig_type=int16  type_size=16  sig_dim=1  device_id=0  sample_time=0.000500
  EtherCAT Rx Var 7 : xpcethercatlib/EtherCAT PDO Receive  Priority=2  sig_name=Box 3 (ATRIAS 2.1 Leg (Medulla 1.5)).Measured Current.Amp 2 Measured Current  sig_offset=1672  sig_type=int16  type_size=16  sig_dim=1  device_id=0  sample_time=0.000500
  EtherCAT Rx Var 8 : xpcethercatlib/EtherCAT PDO Receive  Priority=2  sig_name=Box 3 (ATRIAS 2.1 Leg (Medulla 1.5)).Motor Encoder.Motor Encoder  sig_offset=1400  sig_type=uint32  type_size=32  sig_dim=1  device_id=0  sample_time=0.000500
  EtherCAT Rx Var 9 : xpcethercatlib/EtherCAT PDO Receive  Priority=2  sig_name=Box 3 (ATRIAS 2.1 Leg (Medulla 1.5)).Motor Encoder.Motor Encoder Timestamp  sig_offset=1432  sig_type=uint16  type_size=16  sig_dim=1  device_id=0  sample_time=0.000500
  EtherCAT Tx Var 3 : xpcethercatlib/EtherCAT PDO Transmit   Priority=3  sig_name=Box 3 (ATRIAS 2.1 Leg (Medulla 1.5)).uControllerInput.Command  sig_offset=1344  sig_type=uint8  type_size=8  sig_dim=1  device_id=0  sample_time=0.000500
  EtherCAT Tx Var 4 : xpcethercatlib/EtherCAT PDO Transmit   Priority=3  sig_name=Box 3 (ATRIAS 2.1 Leg (Medulla 1.5)).uControllerInput.Counter  sig_offset=1352  sig_type=uint16  type_size=16  sig_dim=1  device_id=0  sample_time=0.000500
  EtherCAT Tx Var 5 : xpcethercatlib/EtherCAT PDO Transmit   Priority=3  sig_name=Box 3 (ATRIAS 2.1 Leg (Medulla 1.5)).uControllerInput.Motor Current  sig_offset=1368  sig_type=int32  type_size=32  sig_dim=1  device_id=0  sample_time=0.000500
  Mux1 : Mux  Inputs=2
  Mux2 : Mux  Inputs=2
  Mux5 : Mux  Inputs=6
  LegEncoder : Outport
  MotorEncoder : Outport  Port=2
  ToeSensor : Outport  Port=3
  LimitSwitch : Outport  Port=4
  ID : Outport  Port=5
  State : Outport  Port=6
  Counter : Outport  Port=7
  ErrorFlags : Outport  Port=8
  IncEncoder : Outport  Port=9
  LegEncoderTimestamp : Outport  Port=10
  MotorEncoderTimestamp : Outport  Port=11
  IncEncoderTimestamp : Outport  Port=12
  MotorVoltage : Outport  Port=13
  LogicVoltage : Outport  Port=14
  Thermistors : Outport  Port=15
  AmpMeasuredCurrent : Outport  Port=16
  KneeForce : Outport  Port=17
  wires:
  Data Type Conversion3/1 -> EtherCAT Tx Var 3/1
  Data Type Conversion4/1 -> EtherCAT Tx Var 4/1
  Data Type Conversion5/1 -> EtherCAT Tx Var 5/1
  "EtherCAT Rx Var "/1 -> IncEncoder/1
  EtherCAT Rx Var 1/1 -> IncEncoderTimestamp/1
  EtherCAT Rx Var 2/1 -> Mux2/1
  EtherCAT Rx Var 3/1 -> Mux2/2
  EtherCAT Rx Var 4/1 -> LegEncoder/1
  EtherCAT Rx Var 5/1 -> LegEncoderTimestamp/1
  EtherCAT Rx Var 6/1 -> Mux1/1
  EtherCAT Rx Var 7/1 -> Mux1/2
  EtherCAT Rx Var 8/1 -> MotorEncoder/1
  EtherCAT Rx Var 9/1 -> MotorEncoderTimestamp/1
  EtherCAT Rx Var 10/1 -> LogicVoltage/1
  EtherCAT Rx Var 11/1 -> MotorVoltage/1
  EtherCAT Rx Var 12/1 -> Mux5/1
  EtherCAT Rx Var 13/1 -> Mux5/2
  EtherCAT Rx Var 14/1 -> Mux5/3
  EtherCAT Rx Var 15/1 -> Mux5/4
  EtherCAT Rx Var 16/1 -> Mux5/5
  EtherCAT Rx Var 17/1 -> Mux5/6
  EtherCAT Rx Var 18/1 -> Counter/1
  EtherCAT Rx Var 19/1 -> ErrorFlags/1
  EtherCAT Rx Var 20/1 -> ID/1
  EtherCAT Rx Var 21/1 -> LimitSwitch/1
  EtherCAT Rx Var 22/1 -> State/1
  EtherCAT Rx Var 23/1 -> ToeSensor/1
  MedullaCmd/1 -> Data Type Conversion3/1
  MedullaCounter/1 -> Data Type Conversion4/1
  MotorCmd/1 -> Data Type Conversion5/1
  Mux5/1 -> Thermistors/1
  Mux1/1 -> AmpMeasuredCurrent/1
  Mux2/1 -> KneeForce/1

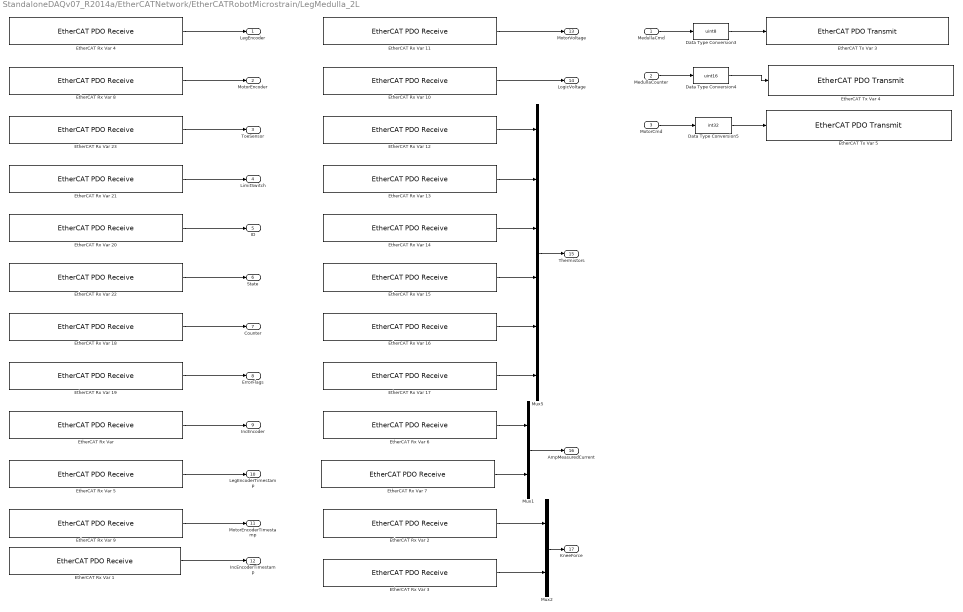
== system StandaloneDAQv07_R2014a/EtherCATNetwork/EtherCATRobotMicrostrain/LegMedulla_2L ==
  MedullaCmd : Inport
  MedullaCounter : Inport  Port=2
  MotorCmd : Inport  Port=3
  Data Type Conversion3 : DataTypeConversion  OutDataTypeStr=uint8  RndMeth=Simplest
  Data Type Conversion4 : DataTypeConversion  OutDataTypeStr=uint16  RndMeth=Simplest
  Data Type Conversion5 : DataTypeConversion  OutDataTypeStr=int32  RndMeth=Simplest
  "EtherCAT Rx Var " : xpcethercatlib/EtherCAT PDO Receive  Priority=2  sig_name=Box 2 (ATRIAS 2.1 Leg (Medulla 1.5)).Incremental Encoder.Incremental Encoder  sig_offset=1120  sig_type=uint16  type_size=16  sig_dim=1  device_id=0  sample_time=0.000500
  EtherCAT Rx Var 1 : xpcethercatlib/EtherCAT PDO Receive  Priority=2  sig_name=Box 2 (ATRIAS 2.1 Leg (Medulla 1.5)).Incremental Encoder.Incremental Encoder Timestamp  sig_offset=1136  sig_type=uint16  type_size=16  sig_dim=1  device_id=0  sample_time=0.000500
  EtherCAT Rx Var 10 : xpcethercatlib/EtherCAT PDO Receive  Priority=2  sig_name=Box 2 (ATRIAS 2.1 Leg (Medulla 1.5)).Power.Logic Voltage  sig_offset=1168  sig_type=uint16  type_size=16  sig_dim=1  device_id=0  sample_time=0.000500
  EtherCAT Rx Var 11 : xpcethercatlib/EtherCAT PDO Receive  Priority=2  sig_name=Box 2 (ATRIAS 2.1 Leg (Medulla 1.5)).Power.Motor Voltage  sig_offset=1152  sig_type=uint16  type_size=16  sig_dim=1  device_id=0  sample_time=0.000500
  EtherCAT Rx Var 12 : xpcethercatlib/EtherCAT PDO Receive  Priority=2  sig_name=Box 2 (ATRIAS 2.1 Leg (Medulla 1.5)).Thermistors.Thermistor 0  sig_offset=1184  sig_type=uint16  type_size=16  sig_dim=1  device_id=0  sample_time=0.000500
  EtherCAT Rx Var 13 : xpcethercatlib/EtherCAT PDO Receive  Priority=2  sig_name=Box 2 (ATRIAS 2.1 Leg (Medulla 1.5)).Thermistors.Thermistor 1  sig_offset=1200  sig_type=uint16  type_size=16  sig_dim=1  device_id=0  sample_time=0.000500
  EtherCAT Rx Var 14 : xpcethercatlib/EtherCAT PDO Receive  Priority=2  sig_name=Box 2 (ATRIAS 2.1 Leg (Medulla 1.5)).Thermistors.Thermistor 2  sig_offset=1216  sig_type=uint16  type_size=16  sig_dim=1  device_id=0  sample_time=0.000500
  EtherCAT Rx Var 15 : xpcethercatlib/EtherCAT PDO Receive  Priority=2  sig_name=Box 2 (ATRIAS 2.1 Leg (Medulla 1.5)).Thermistors.Thermistor 3  sig_offset=1232  sig_type=uint16  type_size=16  sig_dim=1  device_id=0  sample_time=0.000500
  EtherCAT Rx Var 16 : xpcethercatlib/EtherCAT PDO Receive  Priority=2  sig_name=Box 2 (ATRIAS 2.1 Leg (Medulla 1.5)).Thermistors.Thermistor 4  sig_offset=1248  sig_type=uint16  type_size=16  sig_dim=1  device_id=0  sample_time=0.000500
  EtherCAT Rx Var 17 : xpcethercatlib/EtherCAT PDO Receive  Priority=2  sig_name=Box 2 (ATRIAS 2.1 Leg (Medulla 1.5)).Thermistors.Thermistor 5  sig_offset=1264  sig_type=uint16  type_size=16  sig_dim=1  device_id=0  sample_time=0.000500
  EtherCAT Rx Var 18 : xpcethercatlib/EtherCAT PDO Receive  Priority=2  sig_name=Box 2 (ATRIAS 2.1 Leg (Medulla 1.5)).uController Status.Counter  sig_offset=984  sig_type=uint8  type_size=8  sig_dim=1  device_id=0  sample_time=0.000500
  EtherCAT Rx Var 19 : xpcethercatlib/EtherCAT PDO Receive  Priority=2  sig_name=Box 2 (ATRIAS 2.1 Leg (Medulla 1.5)).uController Status.Error Flags  sig_offset=992  sig_type=uint8  type_size=8  sig_dim=1  device_id=0  sample_time=0.000500
  EtherCAT Rx Var 2 : xpcethercatlib/EtherCAT PDO Receive  Priority=2  sig_name=Box 2 (ATRIAS 2.1 Leg (Medulla 1.5)).Knee Force.Knee Force 1  sig_offset=1312  sig_type=uint16  type_size=16  sig_dim=1  device_id=0  sample_time=0.000500
  EtherCAT Rx Var 20 : xpcethercatlib/EtherCAT PDO Receive  Priority=2  sig_name=Box 2 (ATRIAS 2.1 Leg (Medulla 1.5)).uController Status.ID  sig_offset=968  sig_type=uint8  type_size=8  sig_dim=1  device_id=0  sample_time=0.000500
  EtherCAT Rx Var 21 : xpcethercatlib/EtherCAT PDO Receive  Priority=2  sig_name=Box 2 (ATRIAS 2.1 Leg (Medulla 1.5)).uController Status.Limit Switch  sig_offset=1000  sig_type=uint8  type_size=8  sig_dim=1  device_id=0  sample_time=0.000500
  EtherCAT Rx Var 22 : xpcethercatlib/EtherCAT PDO Receive  Priority=2  sig_name=Box 2 (ATRIAS 2.1 Leg (Medulla 1.5)).uController Status.State  sig_offset=976  sig_type=uint8  type_size=8  sig_dim=1  device_id=0  sample_time=0.000500
  EtherCAT Rx Var 23 : xpcethercatlib/EtherCAT PDO Receive  Priority=2  sig_name=Box 2 (ATRIAS 2.1 Leg (Medulla 1.5)).uController Status.Toe Sensor  sig_offset=1008  sig_type=uint16  type_size=16  sig_dim=1  device_id=0  sample_time=0.000500
  EtherCAT Rx Var 3 : xpcethercatlib/EtherCAT PDO Receive  Priority=2  sig_name=Box 2 (ATRIAS 2.1 Leg (Medulla 1.5)).Knee Force.Knee Force 2  sig_offset=1328  sig_type=uint16  type_size=16  sig_dim=1  device_id=0  sample_time=0.000500
  EtherCAT Rx Var 4 : xpcethercatlib/EtherCAT PDO Receive  Priority=2  sig_name=Box 2 (ATRIAS 2.1 Leg (Medulla 1.5)).Leg Encoder.Leg Encoder  sig_offset=1072  sig_type=uint32  type_size=32  sig_dim=1  device_id=0  sample_time=0.000500
  EtherCAT Rx Var 5 : xpcethercatlib/EtherCAT PDO Receive  Priority=2  sig_name=Box 2 (ATRIAS 2.1 Leg (Medulla 1.5)).Leg Encoder.Leg Encoder Timestamp  sig_offset=1104  sig_type=uint16  type_size=16  sig_dim=1  device_id=0  sample_time=0.000500
  EtherCAT Rx Var 6 : xpcethercatlib/EtherCAT PDO Receive  Priority=2  sig_name=Box 2 (ATRIAS 2.1 Leg (Medulla 1.5)).Measured Current.Amp 1 Measured Current  sig_offset=1280  sig_type=int16  type_size=16  sig_dim=1  device_id=0  sample_time=0.000500
  EtherCAT Rx Var 7 : xpcethercatlib/EtherCAT PDO Receive  Priority=2  sig_name=Box 2 (ATRIAS 2.1 Leg (Medulla 1.5)).Measured Current.Amp 2 Measured Current  sig_offset=1296  sig_type=int16  type_size=16  sig_dim=1  device_id=0  sample_time=0.000500
  EtherCAT Rx Var 8 : xpcethercatlib/EtherCAT PDO Receive  Priority=2  sig_name=Box 2 (ATRIAS 2.1 Leg (Medulla 1.5)).Motor Encoder.Motor Encoder  sig_offset=1024  sig_type=uint32  type_size=32  sig_dim=1  device_id=0  sample_time=0.000500
  EtherCAT Rx Var 9 : xpcethercatlib/EtherCAT PDO Receive  Priority=2  sig_name=Box 2 (ATRIAS 2.1 Leg (Medulla 1.5)).Motor Encoder.Motor Encoder Timestamp  sig_offset=1056  sig_type=uint16  type_size=16  sig_dim=1  device_id=0  sample_time=0.000500
  EtherCAT Tx Var 3 : xpcethercatlib/EtherCAT PDO Transmit   Priority=3  sig_name=Box 2 (ATRIAS 2.1 Leg (Medulla 1.5)).uControllerInput.Command  sig_offset=968  sig_type=uint8  type_size=8  sig_dim=1  device_id=0  sample_time=0.000500
  EtherCAT Tx Var 4 : xpcethercatlib/EtherCAT PDO Transmit   Priority=3  sig_name=Box 2 (ATRIAS 2.1 Leg (Medulla 1.5)).uControllerInput.Counter  sig_offset=976  sig_type=uint16  type_size=16  sig_dim=1  device_id=0  sample_time=0.000500
  EtherCAT Tx Var 5 : xpcethercatlib/EtherCAT PDO Transmit   Priority=3  sig_name=Box 2 (ATRIAS 2.1 Leg (Medulla 1.5)).uControllerInput.Motor Current  sig_offset=992  sig_type=int32  type_size=32  sig_dim=1  device_id=0  sample_time=0.000500
  Mux1 : Mux  Inputs=2
  Mux2 : Mux  Inputs=2
  Mux5 : Mux  Inputs=6
  LegEncoder : Outport
  MotorEncoder : Outport  Port=2
  ToeSensor : Outport  Port=3
  LimitSwitch : Outport  Port=4
  ID : Outport  Port=5
  State : Outport  Port=6
  Counter : Outport  Port=7
  ErrorFlags : Outport  Port=8
  IncEncoder : Outport  Port=9
  LegEncoderTimestamp : Outport  Port=10
  MotorEncoderTimestamp : Outport  Port=11
  IncEncoderTimestamp : Outport  Port=12
  MotorVoltage : Outport  Port=13
  LogicVoltage : Outport  Port=14
  Thermistors : Outport  Port=15
  AmpMeasuredCurrent : Outport  Port=16
  KneeForce : Outport  Port=17
  wires:
  Data Type Conversion3/1 -> EtherCAT Tx Var 3/1
  Data Type Conversion4/1 -> EtherCAT Tx Var 4/1
  Data Type Conversion5/1 -> EtherCAT Tx Var 5/1
  "EtherCAT Rx Var "/1 -> IncEncoder/1
  EtherCAT Rx Var 1/1 -> IncEncoderTimestamp/1
  EtherCAT Rx Var 2/1 -> Mux2/1
  EtherCAT Rx Var 3/1 -> Mux2/2
  EtherCAT Rx Var 4/1 -> LegEncoder/1
  EtherCAT Rx Var 5/1 -> LegEncoderTimestamp/1
  EtherCAT Rx Var 6/1 -> Mux1/1
  EtherCAT Rx Var 7/1 -> Mux1/2
  EtherCAT Rx Var 8/1 -> MotorEncoder/1
  EtherCAT Rx Var 9/1 -> MotorEncoderTimestamp/1
  EtherCAT Rx Var 10/1 -> LogicVoltage/1
  EtherCAT Rx Var 11/1 -> MotorVoltage/1
  EtherCAT Rx Var 12/1 -> Mux5/1
  EtherCAT Rx Var 13/1 -> Mux5/2
  EtherCAT Rx Var 14/1 -> Mux5/3
  EtherCAT Rx Var 15/1 -> Mux5/4
  EtherCAT Rx Var 16/1 -> Mux5/5
  EtherCAT Rx Var 17/1 -> Mux5/6
  EtherCAT Rx Var 18/1 -> Counter/1
  EtherCAT Rx Var 19/1 -> ErrorFlags/1
  EtherCAT Rx Var 20/1 -> ID/1
  EtherCAT Rx Var 21/1 -> LimitSwitch/1
  EtherCAT Rx Var 22/1 -> State/1
  EtherCAT Rx Var 23/1 -> ToeSensor/1
  MedullaCmd/1 -> Data Type Conversion3/1
  MedullaCounter/1 -> Data Type Conversion4/1
  MotorCmd/1 -> Data Type Conversion5/1
  Mux5/1 -> Thermistors/1
  Mux1/1 -> AmpMeasuredCurrent/1
  Mux2/1 -> KneeForce/1

== matlab function StandaloneDAQv07_R2014a/SerialInterfaces/KVH/UpdateOrientation/EstimateOrientation ==
  data: DeltaAngle input; Acceleration input; Status input; Sequence input; Reset input; Rk output; wk output; Rkm1 input; wkm1 input; Akm1 input; Ak output; Seqkm1 input; Seqk output
function [Rk, wk, Ak, Seqk] = fcn(DeltaAngle,Acceleration,Status,Sequence,Reset,Rkm1,wkm1,Akm1,Seqkm1) %#codegen
    [Rk, wk, Ak, Seqk] = estimateOrientation(DeltaAngle,Acceleration,Rkm1,wkm1,Akm1,Status,Sequence,Seqkm1,Reset);
end

== matlab function StandaloneDAQv07_R2014a/SerialInterfaces/KVH/UpdateOrientation/MATLAB Function ==
  data: P input; Rotation output; Acceleration output; Status output; Sequence output; Temperature output; Valid output
function [Rotation,Acceleration,Status,Sequence,Temperature,Valid] = KVHParsePacket(P)
    %#codegen
    CMD = [254; 129; 255; 85]; %hex2dec(['FE';'81';'FF';'55']);
    
    Valid = false;
    if all(P(1:4) == CMD)
        Valid = kvhCheckCRC(P(1:36));
    end
    
    Rotation = parseSingle(P(5:16,:));
    Acceleration = parseSingle(P(17:28,:));
    Status = P(29);
    Sequence = double(P(30));
    Temperature = parseInt16(P(31:32));
end

function S = parseSingle(D)
    Stmp1 = uint32(reshape(D,4,[]));
    Stmp2 = 16777216*Stmp1(1,:) + 65536*Stmp1(2,:) + 256*Stmp1(3,:) + Stmp1(4,:);
    Stmp3 = typecast(Stmp2,'single');
    S = double(Stmp3');
end

function S = parseInt16(D)
    Stmp1 = uint16(reshape(D,2,[]));
    Stmp2 = 256*Stmp1(1,:) + Stmp1(2,:);
    S = double(Stmp2');
end

== matlab function StandaloneDAQv07_R2014a/EtherCATNetwork/EtherCATRobotMicrostrain/IMU_Medulla/TypecastAndCast2 ==
  data: u input uint32; y output
function y = unit32_to_double(u)
    %#codegen
    ys = typecast(u, 'single');
    y  = double(ys);
end
